simulink model "Task15"  (R2019b)
settings: Solver=VariableStepAuto  StartTime=0.0  StopTime=10.0  RelTol=1e-3
settings Model: Creator=12393  LastModifiedBy=12393

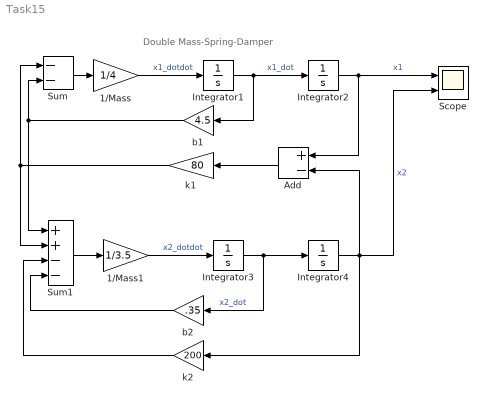
== system Task15 ==
  note: Double Mass-Spring-Damper
  1/Mass : Gain  Gain=1/4  SaturateOnIntegerOverflow=on  OutDataTypeStr=Inherit: Same as input  ParamDataTypeStr=Inherit: Same as input
  1/Mass1 : Gain  Gain=1/3.5  SaturateOnIntegerOverflow=on  OutDataTypeStr=Inherit: Same as input  ParamDataTypeStr=Inherit: Same as input
  Add : Sum  Inputs=+-
  Integrator1 : Integrator
  Integrator2 : Integrator  InitialCondition=4
      settings: AttributesFormatString=x1(0) = %<InitialCondition> m
  Integrator3 : Integrator
  Integrator4 : Integrator  InitialCondition=2
      settings: AttributesFormatString=x2(0) = %<InitialCondition> m
  Scope : Scope  NumInputPorts=2
  Sum : Sum  Inputs=--  SaturateOnIntegerOverflow=on  InputSameDT=on  OutDataTypeStr=Inherit: Same as first input
  Sum1 : Sum  Inputs=++--  SaturateOnIntegerOverflow=on  InputSameDT=on  OutDataTypeStr=Inherit: Same as first input
  b1 : Gain  Gain=4.5  SaturateOnIntegerOverflow=on  OutDataTypeStr=Inherit: Same as input  ParamDataTypeStr=Inherit: Same as input
  b2 : Gain  Gain=.35  SaturateOnIntegerOverflow=on  OutDataTypeStr=Inherit: Same as input  ParamDataTypeStr=Inherit: Same as input
  k1 : Gain  Gain=80  SaturateOnIntegerOverflow=on  OutDataTypeStr=Inherit: Same as input  ParamDataTypeStr=Inherit: Same as input
  k2 : Gain  Gain=200  SaturateOnIntegerOverflow=on  OutDataTypeStr=Inherit: Same as input  ParamDataTypeStr=Inherit: Same as input
  wires:
  1/Mass1/1 -> Integrator3/1  "x2_dotdot"
  b2/1 -> Sum1/4
  Integrator4/1 -> Add/2, Scope/2, k2/1  "x2"
  k2/1 -> Sum1/3
  Sum1/1 -> 1/Mass1/1
  Add/1 -> k1/1
  b1/1 -> Sum/2, Sum1/1
  Integrator1/1 -> Integrator2/1, b1/1  "x1_dot"
  k1/1 -> Sum/1, Sum1/2
  1/Mass/1 -> Integrator1/1  "x1_dotdot"
  Sum/1 -> 1/Mass/1
  Integrator2/1 -> Scope/1, Add/1  "x1"
  Integrator3/1 -> Integrator4/1, b2/1  "x2_dot"
